simulink model "MISO_test1"  (R2023b)
settings: Solver=VariableStepAuto  StartTime=0.0  StopTime=0.001  RelTol=1e-3
libraries: spsSeriesRLCBranchLib x8, spsDiodeLib x4, spsIGBTLib x4, spsPVArrayLib x4, spsVoltageMeasurementLib x2, sps_lib x1
settings Model: Creator=JAZXII  LastModifiedBy=JAZXII

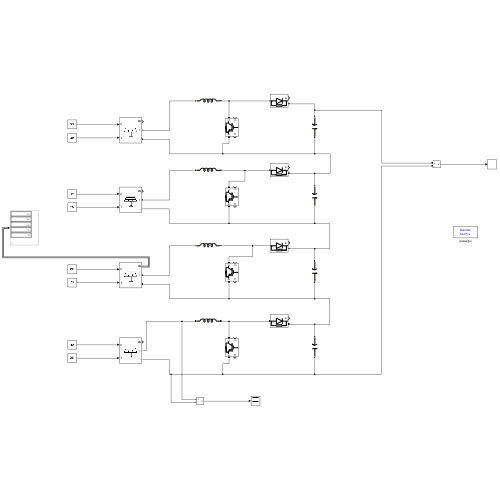
[thumbnail: Simulink's stored preview of the top-level diagram]
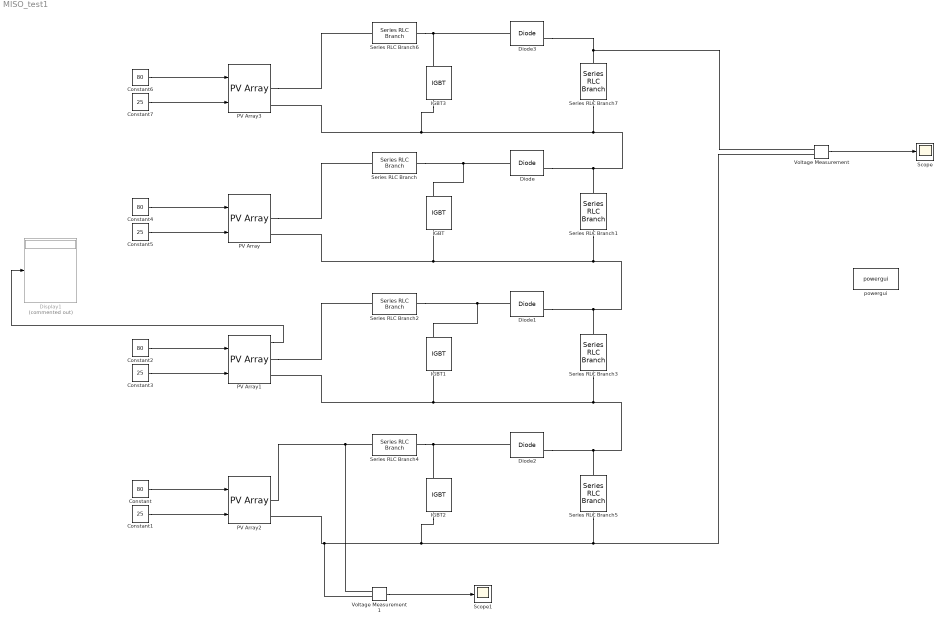
== system MISO_test1 ==
  Constant{,2,4,6} (4 alike) : Constant  Value=80
  Constant{1,3,5,7} (4 alike) : Constant  Value=25
  Diode{,1..3} (4 alike) : spsDiodeLib/Diode  Ron=0.001  Lon=0  Vf=0.8  IC=0  UseSnubber=0  Rs=500  Cs=250e-9  Measurements=on
  Display1 : Display  Commented=on
  IGBT{,1..3} (4 alike) : spsIGBTLib/IGBT  Ron=0.001  Lon=0  Vf=1  Tf=1e-6  Tt=2e-6  IC=0  Rs=1e5  Cs=inf  Measurements=on
  PV Array : spsPVArrayLib/PV Array  Npar=2  Nser=10  PlotType=array @ 1000 W/m2 & specified temperatures  S_vec="[ 1000  500  100 ]"  Temp_C_vec="[ 45 25  ]"  ModuleName=User-defined  PlotWhenSelected=off  Pm=22.05  Ncell=10  Voc=36.3  Isc=7.84  Vm=3  Im=7.35  beta_Voc_pc=-0.36099  alpha_Isc_pc=0.102  beta_Voc=-0.13104  alpha_Isc=0.0079968  IL=7.9183  I0=1.5749e-15  nI=2.9999  Rsh=12.2453  Rs=0.00054238  RobustModel=off  RobustCellTemperature=313.3991  BAL=on  Tc=1e-6  Tfilter=5e-5
  PV Array1 : spsPVArrayLib/PV Array  Npar=2  Nser=10  PlotType=array @ 1000 W/m2 & specified temperatures  S_vec="[ 1000  500  100 ]"  Temp_C_vec="[ 45 25  ]"  ModuleName=User-defined  PlotWhenSelected=off  Pm=22.05  Ncell=10  Voc=36.3  Isc=7.84  Vm=3  Im=7.35  beta_Voc_pc=-0.36099  alpha_Isc_pc=0.102  beta_Voc=-0.13104  alpha_Isc=0.0079968  IL=7.9183  I0=1.5749e-15  nI=2.9999  Rsh=12.2453  Rs=0.00054238  RobustModel=off  RobustCellTemperature=313.3991  BAL=on  Tc=1e-6  Tfilter=5e-5
  PV Array2 : spsPVArrayLib/PV Array  Npar=2  Nser=10  PlotType=array @ 1000 W/m2 & specified temperatures  S_vec="[ 1000  500  100 ]"  Temp_C_vec="[ 45 25  ]"  ModuleName=User-defined  PlotWhenSelected=off  Pm=22.05  Ncell=10  Voc=36.3  Isc=7.84  Vm=3  Im=7.35  beta_Voc_pc=-0.36099  alpha_Isc_pc=0.102  beta_Voc=-0.13104  alpha_Isc=0.0079968  IL=7.9183  I0=1.5749e-15  nI=2.9999  Rsh=12.2453  Rs=0.00054238  RobustModel=off  RobustCellTemperature=313.3991  BAL=on  Tc=1e-6  Tfilter=5e-5
  PV Array3 : spsPVArrayLib/PV Array  Npar=5  Nser=10  PlotType=array @ 1000 W/m2 & specified temperatures  S_vec="[ 1000  500  100 ]"  Temp_C_vec="[ 45 25  ]"  ModuleName=User-defined  PlotWhenSelected=off  Pm=22.05  Ncell=10  Voc=36.3  Isc=7.84  Vm=3  Im=7.35  beta_Voc_pc=-0.36099  alpha_Isc_pc=0.102  beta_Voc=-0.13104  alpha_Isc=0.0079968  IL=7.9183  I0=1.5749e-15  nI=2.9999  Rsh=12.2453  Rs=0.00054238  RobustModel=off  RobustCellTemperature=313.3991  BAL=on  Tc=1e-6  Tfilter=5e-5
  Scope : Scope
  Scope1 : Scope
  Series RLC Branch{,2,4,6} (4 alike) : spsSeriesRLCBranchLib/Series RLC Branch  LConnTagsString=__new0  RConnTagsString=__new0  BranchType=L  Resistance=1  Inductance=7.875  SetiL0=off  InitialCurrent=0  Capacitance=1e-6  Setx0=off  InitialVoltage=0  Measurements=None
  Series RLC Branch{1,3,5,7} (4 alike) : spsSeriesRLCBranchLib/Series RLC Branch  LConnTagsString=__new0  RConnTagsString=__new0  BranchType=C  Resistance=1  Inductance=1e-3  SetiL0=off  InitialCurrent=0  Capacitance=2.986  Setx0=off  InitialVoltage=0  Measurements=None
  Voltage Measurement : spsVoltageMeasurementLib/Voltage Measurement  PhasorSimulation=off  OutputType=Complex  PSBequivalent=0
  Voltage Measurement1 : spsVoltageMeasurementLib/Voltage Measurement  PhasorSimulation=off  OutputType=Complex  PSBequivalent=0
  powergui : sps_lib/powergui  Priority=1  SimulationMode=Discrete  SampleTime=50e-6  frequency=60  Iterations=50  frequencyindice=0  Pbase=100e6  ErrMax=1e-4  UnitsV=kV  UnitsW=MW  buscounter=0  FunctionMessages=off  echomessages=off  EnableUseOfTLC=off  CurrentSourceSwitches=off  DisableSnubberDevices=off  DisableRonSwitches=off  DisableVfSwitches=off  DisplayEquations=off  AutomaticDiscreteSolvers=off  SolverType=Tustin/Backward Euler (TBE)  Interpol=off  ExternalGateDelay=off  methode=off  Ts=100  x0status=blocks  SPID=on  SwTol=0  HookPort=off  NonlinearTolerance=1e-4  nMaxIteration=100  ContinueOnMaxIteration=off  RestoreLinks=warning  ResistiveCurrentMeasurement=off  Frange=[0:2:500]  Ylog=off  Xlog=on  ShowGrid=off  save=off  variable=ZData  structure=0  ZoomFFT=off  StartTime=0.0  cycles=1  DisplayStyle=1  fundamental=60  FreqAxis=off  MaxFrequency=1000  frequencyindicesteady=1  RmsSteady=1  display=off
  wires:
  Voltage Measurement/1 -> Scope/1
  Voltage Measurement1/1 -> Scope1/1
  Constant/1 -> PV Array2/1
  Constant1/1 -> PV Array2/2
  Constant6/1 -> PV Array3/1
  Constant7/1 -> PV Array3/2
  Constant4/1 -> PV Array/1
  Constant5/1 -> PV Array/2
  Constant2/1 -> PV Array1/1
  Constant3/1 -> PV Array1/2
  PV Array1/1 -> Display1/1
  connections:
  PV Array/RConn1 -- Series RLC Branch/LConn1
  Series RLC Branch/RConn1 -- IGBT/LConn1 -- Diode/LConn1
  Series RLC Branch1/LConn1 -- PV Array/RConn2 -- IGBT/RConn1 -- Diode1/RConn1 -- Series RLC Branch3/RConn1
  Series RLC Branch3/LConn1 -- Series RLC Branch5/RConn1 -- Diode2/RConn1 -- PV Array1/RConn2 -- IGBT1/RConn1
  Series RLC Branch2/RConn1 -- IGBT1/LConn1 -- Diode1/LConn1
  PV Array1/RConn1 -- Series RLC Branch2/LConn1
  Voltage Measurement/LConn2 -- Series RLC Branch5/LConn1 -- IGBT2/RConn1 -- Voltage Measurement1/LConn2 -- PV Array2/RConn2
  Series RLC Branch4/RConn1 -- Diode2/LConn1 -- IGBT2/LConn1
  Voltage Measurement1/LConn1 -- Series RLC Branch4/LConn1 -- PV Array2/RConn1
  Series RLC Branch6/RConn1 -- Diode3/LConn1 -- IGBT3/LConn1
  Series RLC Branch1/RConn1 -- Diode/RConn1 -- Series RLC Branch7/LConn1 -- IGBT3/RConn1 -- PV Array3/RConn2
  Diode3/RConn1 -- Voltage Measurement/LConn1 -- Series RLC Branch7/RConn1
  PV Array3/RConn1 -- Series RLC Branch6/LConn1
